simulink model "ctrl_student_HIL"  (R2015a)
settings: Solver=ode4  StartTime=0.0  StopTime=inf  FixedStep=0.01  RelTol=1e-3
(part 1 of 3)
settings Model: CovSFcnEnable=off  Creator=mclab  LastModifiedBy=MCLab
settings DebuggingCC: SolverPrmCheckMsg=warning  InheritedTsInSrcMsg=none
settings RTWCC: SystemTargetFile=NIVeriStand_VxWorks.tlc  TemplateMakefile=NIVeriStand_VxWorks.tmf  Description=NI VeriStand VxWorks Real-Time Target for Release 2007b or later
settings STFCustomTargetCC: GenerateSampleERTMain=off  GeneratePreprocessorConditionals=Disable all  ERTCustomFileBanners=off  MatFileLogging=on  SupportNonInlinedSFcns=on  SupportVariableSizeSignals=off  MATLABClassNameForMDSCustomization=Simulink.SoftwareTarget.TargetSpecificTriggerConfigurationBase  GRTInterface=on  SystemTargetFile=NIVeriStand_VxWorks.tlc

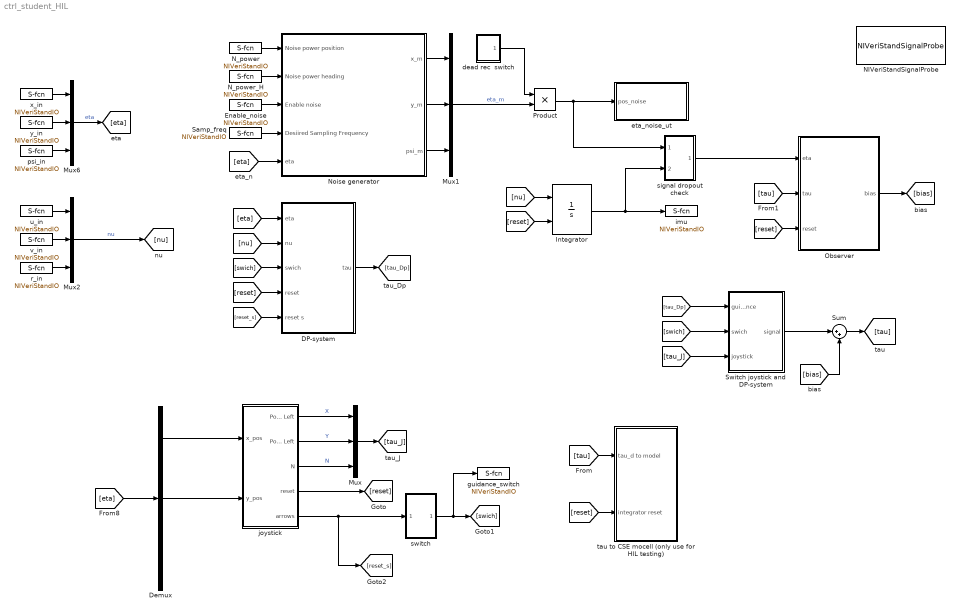
== system ctrl_student_HIL ==
  DP-system : Subsystem
  Demux : Demux  Outputs=3
  Enable_noise : S-Function  Priority=10  FunctionName=NIVeriStandIO  Parameters=width dtype portnum stime stype btype  mask(NI VeriStand Inport){portnum=10, width=-1, stime=-1, dtype=auto, stype=auto, btype=1}
      mask prompts: portnum "Port number:"; width "Port dimensions (-1 for dynamically sized):"; stime "Sample time (-1 for inherited):"; dtype "Data type:"; stype "Signal type:"; btype "Block type:"
      mask help: Use this inport on any level of nested subsystems to allow NI VeriStand software to map signals to it.
      mask init:
      | NIVeriStandIO_init;
      settings: CopyFcn=NIVeriStand_MDL_functions('', 'IO_copy');  DeleteFcn=NIVeriStand_MDL_functions('', 'IO_delete');  MoveFcn=set_param(gcb, 'Mask', 'on');
      mask Callback portnum: NIVeriStand_MDL_functions('', 'IO_setportnum');
      mask TypeOptions dtype: auto | double | single | int8 | uint8 | int16 | uint16 | int32 | uint32 | boolean
      mask Callback dtype: NIVeriStand_MDL_functions('', 'IO_booleansignal');
      mask TypeOptions stype: auto | real | complex
      mask Display:
      | patch([-x x], [-y y], [.90980 .81960 .32156]);
      | plot([xrad -x x xrad], [yrad -y y yrad]);
      | fprintf('NI In%d', portnum);
  Integrator : Integrator  ExternalReset=either
  Mux{,1..2,6} (4 alike) : Mux  Inputs=3
  NIVeriStandSignalProbe : S-Function  FunctionName=NIVeriStandSignalProbe  Parameters=1
  N_power : S-Function  Priority=7  FunctionName=NIVeriStandIO  Parameters=width dtype portnum stime stype btype  mask(NI VeriStand Inport){portnum=7, width=-1, stime=-1, dtype=auto, stype=auto, btype=1}
      mask prompts: portnum "Port number:"; width "Port dimensions (-1 for dynamically sized):"; stime "Sample time (-1 for inherited):"; dtype "Data type:"; stype "Signal type:"; btype "Block type:"
      mask help: Use this inport on any level of nested subsystems to allow NI VeriStand software to map signals to it.
      mask init:
      | NIVeriStandIO_init;
      settings: CopyFcn=NIVeriStand_MDL_functions('', 'IO_copy');  DeleteFcn=NIVeriStand_MDL_functions('', 'IO_delete');  MoveFcn=set_param(gcb, 'Mask', 'on');
      mask Callback portnum: NIVeriStand_MDL_functions('', 'IO_setportnum');
      mask TypeOptions dtype: auto | double | single | int8 | uint8 | int16 | uint16 | int32 | uint32 | boolean
      mask Callback dtype: NIVeriStand_MDL_functions('', 'IO_booleansignal');
      mask TypeOptions stype: auto | real | complex
      mask Display:
      | patch([-x x], [-y y], [.90980 .81960 .32156]);
      | plot([xrad -x x xrad], [yrad -y y yrad]);
      | fprintf('NI In%d', portnum);
  N_power_H : S-Function  Priority=8  FunctionName=NIVeriStandIO  Parameters=width dtype portnum stime stype btype  mask(NI VeriStand Inport){portnum=8, width=-1, stime=-1, dtype=auto, stype=auto, btype=1}
      mask prompts: portnum "Port number:"; width "Port dimensions (-1 for dynamically sized):"; stime "Sample time (-1 for inherited):"; dtype "Data type:"; stype "Signal type:"; btype "Block type:"
      mask help: Use this inport on any level of nested subsystems to allow NI VeriStand software to map signals to it.
      mask init:
      | NIVeriStandIO_init;
      settings: CopyFcn=NIVeriStand_MDL_functions('', 'IO_copy');  DeleteFcn=NIVeriStand_MDL_functions('', 'IO_delete');  MoveFcn=set_param(gcb, 'Mask', 'on');
      mask Callback portnum: NIVeriStand_MDL_functions('', 'IO_setportnum');
      mask TypeOptions dtype: auto | double | single | int8 | uint8 | int16 | uint16 | int32 | uint32 | boolean
      mask Callback dtype: NIVeriStand_MDL_functions('', 'IO_booleansignal');
      mask TypeOptions stype: auto | real | complex
      mask Display:
      | patch([-x x], [-y y], [.90980 .81960 .32156]);
      | plot([xrad -x x xrad], [yrad -y y yrad]);
      | fprintf('NI In%d', portnum);
  Noise generator : Subsystem
  Observer : Subsystem
  Product : Product
  Samp_freq : S-Function  Priority=9  FunctionName=NIVeriStandIO  Parameters=width dtype portnum stime stype btype  mask(NI VeriStand Inport){portnum=9, width=-1, stime=-1, dtype=auto, stype=auto, btype=1}
      mask prompts: portnum "Port number:"; width "Port dimensions (-1 for dynamically sized):"; stime "Sample time (-1 for inherited):"; dtype "Data type:"; stype "Signal type:"; btype "Block type:"
      mask help: Use this inport on any level of nested subsystems to allow NI VeriStand software to map signals to it.
      mask init:
      | NIVeriStandIO_init;
      settings: CopyFcn=NIVeriStand_MDL_functions('', 'IO_copy');  DeleteFcn=NIVeriStand_MDL_functions('', 'IO_delete');  MoveFcn=set_param(gcb, 'Mask', 'on');
      mask Callback portnum: NIVeriStand_MDL_functions('', 'IO_setportnum');
      mask TypeOptions dtype: auto | double | single | int8 | uint8 | int16 | uint16 | int32 | uint32 | boolean
      mask Callback dtype: NIVeriStand_MDL_functions('', 'IO_booleansignal');
      mask TypeOptions stype: auto | real | complex
      mask Display:
      | patch([-x x], [-y y], [.90980 .81960 .32156]);
      | plot([xrad -x x xrad], [yrad -y y yrad]);
      | fprintf('NI In%d', portnum);
  Sum : Sum  Inputs=|++
  Switch joystick and DP-system : MATLAB Function  TreatAsAtomicUnit=on
  dead rec  switch : Subsystem
  eta_noise_ut : Subsystem
  guidance_switch : S-Function  Priority=2  FunctionName=NIVeriStandIO  Parameters=width dtype portnum stime stype btype  mask(NI VeriStand Outport){portnum=2, width=-1, stime=-1, dtype=auto, stype=auto, btype=0}
      mask prompts: portnum "Port number:"; width "Port dimensions (-1 for dynamically sized):"; stime "Sample time (-1 for inherited):"; dtype "Data type:"; stype "Signal type:"; btype "Block type:"
      mask help: Use this outport on any level of nested subsystems to allow NI VeriStand software to map signals to it.
      mask init:
      | NIVeriStandIO_init;
      settings: CopyFcn=NIVeriStand_MDL_functions('', 'IO_copy');  DeleteFcn=NIVeriStand_MDL_functions('', 'IO_delete');  MoveFcn=set_param(gcb, 'Mask', 'on');
      mask Callback portnum: NIVeriStand_MDL_functions('', 'IO_setportnum');
      mask TypeOptions dtype: auto | double | single | int8 | uint8 | int16 | uint16 | int32 | uint32 | boolean
      mask Callback dtype: NIVeriStand_MDL_functions('', 'IO_booleansignal');
      mask TypeOptions stype: auto | real | complex
      mask Display:
      | patch([-x x], [-y y], [.90980 .81960 .32156]);
      | plot([xrad -x x xrad], [yrad -y y yrad]);
      | fprintf('NI Out%d', portnum);
  imu : S-Function  Priority=1  FunctionName=NIVeriStandIO  Parameters=width dtype portnum stime stype btype  mask(NI VeriStand Outport){portnum=1, width=-1, stime=-1, dtype=auto, stype=auto, btype=0}
      mask prompts: portnum "Port number:"; width "Port dimensions (-1 for dynamically sized):"; stime "Sample time (-1 for inherited):"; dtype "Data type:"; stype "Signal type:"; btype "Block type:"
      mask help: Use this outport on any level of nested subsystems to allow NI VeriStand software to map signals to it.
      mask init:
      | NIVeriStandIO_init;
      settings: CopyFcn=NIVeriStand_MDL_functions('', 'IO_copy');  DeleteFcn=NIVeriStand_MDL_functions('', 'IO_delete');  MoveFcn=set_param(gcb, 'Mask', 'on');
      mask Callback portnum: NIVeriStand_MDL_functions('', 'IO_setportnum');
      mask TypeOptions dtype: auto | double | single | int8 | uint8 | int16 | uint16 | int32 | uint32 | boolean
      mask Callback dtype: NIVeriStand_MDL_functions('', 'IO_booleansignal');
      mask TypeOptions stype: auto | real | complex
      mask Display:
      | patch([-x x], [-y y], [.90980 .81960 .32156]);
      | plot([xrad -x x xrad], [yrad -y y yrad]);
      | fprintf('NI Out%d', portnum);
  joystick : Subsystem
  psi_in : S-Function  Priority=2  FunctionName=NIVeriStandIO  Parameters=width dtype portnum stime stype btype  mask(NI VeriStand Inport){portnum=2, width=-1, stime=-1, dtype=auto, stype=auto, btype=1}
      mask prompts: portnum "Port number:"; width "Port dimensions (-1 for dynamically sized):"; stime "Sample time (-1 for inherited):"; dtype "Data type:"; stype "Signal type:"; btype "Block type:"
      mask help: Use this inport on any level of nested subsystems to allow NI VeriStand software to map signals to it.
      mask init:
      | NIVeriStandIO_init;
      settings: CopyFcn=NIVeriStand_MDL_functions('', 'IO_copy');  DeleteFcn=NIVeriStand_MDL_functions('', 'IO_delete');  MoveFcn=set_param(gcb, 'Mask', 'on');
      mask Callback portnum: NIVeriStand_MDL_functions('', 'IO_setportnum');
      mask TypeOptions dtype: auto | double | single | int8 | uint8 | int16 | uint16 | int32 | uint32 | boolean
      mask Callback dtype: NIVeriStand_MDL_functions('', 'IO_booleansignal');
      mask TypeOptions stype: auto | real | complex
      mask Display:
      | patch([-x x], [-y y], [.90980 .81960 .32156]);
      | plot([xrad -x x xrad], [yrad -y y yrad]);
      | fprintf('NI In%d', portnum);
  r_in : S-Function  Priority=4  FunctionName=NIVeriStandIO  Parameters=width dtype portnum stime stype btype  mask(NI VeriStand Inport){portnum=4, width=-1, stime=-1, dtype=auto, stype=auto, btype=1}
      mask prompts: portnum "Port number:"; width "Port dimensions (-1 for dynamically sized):"; stime "Sample time (-1 for inherited):"; dtype "Data type:"; stype "Signal type:"; btype "Block type:"
      mask help: Use this inport on any level of nested subsystems to allow NI VeriStand software to map signals to it.
      mask init:
      | NIVeriStandIO_init;
      settings: CopyFcn=NIVeriStand_MDL_functions('', 'IO_copy');  DeleteFcn=NIVeriStand_MDL_functions('', 'IO_delete');  MoveFcn=set_param(gcb, 'Mask', 'on');
      mask Callback portnum: NIVeriStand_MDL_functions('', 'IO_setportnum');
      mask TypeOptions dtype: auto | double | single | int8 | uint8 | int16 | uint16 | int32 | uint32 | boolean
      mask Callback dtype: NIVeriStand_MDL_functions('', 'IO_booleansignal');
      mask TypeOptions stype: auto | real | complex
      mask Display:
      | patch([-x x], [-y y], [.90980 .81960 .32156]);
      | plot([xrad -x x xrad], [yrad -y y yrad]);
      | fprintf('NI In%d', portnum);
  "signal dropout check " : Subsystem
  switch : Subsystem
  tau to CSE mocell (only use for HIL testing) : Subsystem
  u_in : S-Function  Priority=5  FunctionName=NIVeriStandIO  Parameters=width dtype portnum stime stype btype  mask(NI VeriStand Inport){portnum=5, width=-1, stime=-1, dtype=auto, stype=auto, btype=1}
      mask prompts: portnum "Port number:"; width "Port dimensions (-1 for dynamically sized):"; stime "Sample time (-1 for inherited):"; dtype "Data type:"; stype "Signal type:"; btype "Block type:"
      mask help: Use this inport on any level of nested subsystems to allow NI VeriStand software to map signals to it.
      mask init:
      | NIVeriStandIO_init;
      settings: CopyFcn=NIVeriStand_MDL_functions('', 'IO_copy');  DeleteFcn=NIVeriStand_MDL_functions('', 'IO_delete');  MoveFcn=set_param(gcb, 'Mask', 'on');
      mask Callback portnum: NIVeriStand_MDL_functions('', 'IO_setportnum');
      mask TypeOptions dtype: auto | double | single | int8 | uint8 | int16 | uint16 | int32 | uint32 | boolean
      mask Callback dtype: NIVeriStand_MDL_functions('', 'IO_booleansignal');
      mask TypeOptions stype: auto | real | complex
      mask Display:
      | patch([-x x], [-y y], [.90980 .81960 .32156]);
      | plot([xrad -x x xrad], [yrad -y y yrad]);
      | fprintf('NI In%d', portnum);
  v_in : S-Function  Priority=6  FunctionName=NIVeriStandIO  Parameters=width dtype portnum stime stype btype  mask(NI VeriStand Inport){portnum=6, width=-1, stime=-1, dtype=auto, stype=auto, btype=1}
      mask prompts: portnum "Port number:"; width "Port dimensions (-1 for dynamically sized):"; stime "Sample time (-1 for inherited):"; dtype "Data type:"; stype "Signal type:"; btype "Block type:"
      mask help: Use this inport on any level of nested subsystems to allow NI VeriStand software to map signals to it.
      mask init:
      | NIVeriStandIO_init;
      settings: CopyFcn=NIVeriStand_MDL_functions('', 'IO_copy');  DeleteFcn=NIVeriStand_MDL_functions('', 'IO_delete');  MoveFcn=set_param(gcb, 'Mask', 'on');
      mask Callback portnum: NIVeriStand_MDL_functions('', 'IO_setportnum');
      mask TypeOptions dtype: auto | double | single | int8 | uint8 | int16 | uint16 | int32 | uint32 | boolean
      mask Callback dtype: NIVeriStand_MDL_functions('', 'IO_booleansignal');
      mask TypeOptions stype: auto | real | complex
      mask Display:
      | patch([-x x], [-y y], [.90980 .81960 .32156]);
      | plot([xrad -x x xrad], [yrad -y y yrad]);
      | fprintf('NI In%d', portnum);
  x_in : S-Function  Priority=3  FunctionName=NIVeriStandIO  Parameters=width dtype portnum stime stype btype  mask(NI VeriStand Inport){portnum=3, width=-1, stime=-1, dtype=auto, stype=auto, btype=1}
      mask prompts: portnum "Port number:"; width "Port dimensions (-1 for dynamically sized):"; stime "Sample time (-1 for inherited):"; dtype "Data type:"; stype "Signal type:"; btype "Block type:"
      mask help: Use this inport on any level of nested subsystems to allow NI VeriStand software to map signals to it.
      mask init:
      | NIVeriStandIO_init;
      settings: CopyFcn=NIVeriStand_MDL_functions('', 'IO_copy');  DeleteFcn=NIVeriStand_MDL_functions('', 'IO_delete');  MoveFcn=set_param(gcb, 'Mask', 'on');
      mask Callback portnum: NIVeriStand_MDL_functions('', 'IO_setportnum');
      mask TypeOptions dtype: auto | double | single | int8 | uint8 | int16 | uint16 | int32 | uint32 | boolean
      mask Callback dtype: NIVeriStand_MDL_functions('', 'IO_booleansignal');
      mask TypeOptions stype: auto | real | complex
      mask Display:
      | patch([-x x], [-y y], [.90980 .81960 .32156]);
      | plot([xrad -x x xrad], [yrad -y y yrad]);
      | fprintf('NI In%d', portnum);
  y_in : S-Function  Priority=1  FunctionName=NIVeriStandIO  Parameters=width dtype portnum stime stype btype  mask(NI VeriStand Inport){portnum=1, width=-1, stime=-1, dtype=auto, stype=auto, btype=1}
      mask prompts: portnum "Port number:"; width "Port dimensions (-1 for dynamically sized):"; stime "Sample time (-1 for inherited):"; dtype "Data type:"; stype "Signal type:"; btype "Block type:"
      mask help: Use this inport on any level of nested subsystems to allow NI VeriStand software to map signals to it.
      mask init:
      | NIVeriStandIO_init;
      settings: CopyFcn=NIVeriStand_MDL_functions('', 'IO_copy');  DeleteFcn=NIVeriStand_MDL_functions('', 'IO_delete');  MoveFcn=set_param(gcb, 'Mask', 'on');
      mask Callback portnum: NIVeriStand_MDL_functions('', 'IO_setportnum');
      mask TypeOptions dtype: auto | double | single | int8 | uint8 | int16 | uint16 | int32 | uint32 | boolean
      mask Callback dtype: NIVeriStand_MDL_functions('', 'IO_booleansignal');
      mask TypeOptions stype: auto | real | complex
      mask Display:
      | patch([-x x], [-y y], [.90980 .81960 .32156]);
      | plot([xrad -x x xrad], [yrad -y y yrad]);
      | fprintf('NI In%d', portnum);
  wires:
  joystick/3(N) -> Mux/3  "N"
  x_in/1 -> Mux6/1
  y_in/1 -> Mux6/2
  psi_in/1 -> Mux6/3
  Noise generator/1(x_m) -> Mux1/1
  Noise generator/2(y_m) -> Mux1/2
  Noise generator/3(psi_m) -> Mux1/3
  joystick/2(PosY Left) -> Mux/2  "Y"
  joystick/1(PosX Left) -> Mux/1  "X"
  u_in/1 -> Mux2/1
  v_in/1 -> Mux2/2
  r_in/1 -> Mux2/3
  Samp_freq/1 -> Noise generator/4(Desiired Sampling Frequency)
  Enable_noise/1 -> Noise generator/3(Enable noise)
  N_power_H/1 -> Noise generator/2(Noise power heading)
  N_power/1 -> Noise generator/1(Noise power position)
  Mux1/1 -> Product/2  "eta_m"
  Product/1 -> eta_noise_ut/1(pos_noise), "signal dropout check "/1(eta_n)
  dead rec  switch/1(Out1) -> Product/1
  "signal dropout check "/1(eta) -> Observer/1(eta)
  joystick/4(reset) -> [reset]
  [reset] -> Observer/3(reset)
  [reset] -> tau to CSE mocell (only use for HIL testing)/2(integrator reset)
  Integrator/1 -> imu/1, "signal dropout check "/2(imu)
  [reset] -> Integrator/2
  joystick/5(arrows) -> [reset_s], switch/1(In1)
  switch/1(Out1) -> guidance_switch/1, [swich]
  [swich] -> DP-system/3(swich)
  [swich] -> Switch joystick and DP-system/2(swich)
  [reset] -> DP-system/4("reset ")
  [reset_s] -> DP-system/5(reset s)
  [eta] -> Noise generator/5(eta)
  [eta] -> DP-system/1(eta)
  [eta] -> Demux/1
  Demux/1 -> joystick/1(x_pos)
  Demux/2 -> joystick/2(y_pos)
  Mux6/1 -> [eta]  "eta"
  Mux2/1 -> [nu]  "nu"
  [nu] -> DP-system/2(nu)
  [nu] -> Integrator/1
  DP-system/1(tau) -> [tau_Dp]
  [tau_Dp] -> Switch joystick and DP-system/1(guidance)
  Mux/1 -> [tau_J]
  [tau_J] -> Switch joystick and DP-system/3(joystick)
  [tau] -> Observer/2(tau)
  [tau] -> tau to CSE mocell (only use for HIL testing)/1(tau_d to model)
  Observer/1(bias) -> [bias]
  Switch joystick and DP-system/1(signal) -> Sum/1
  [bias] -> Sum/2
  Sum/1 -> [tau]

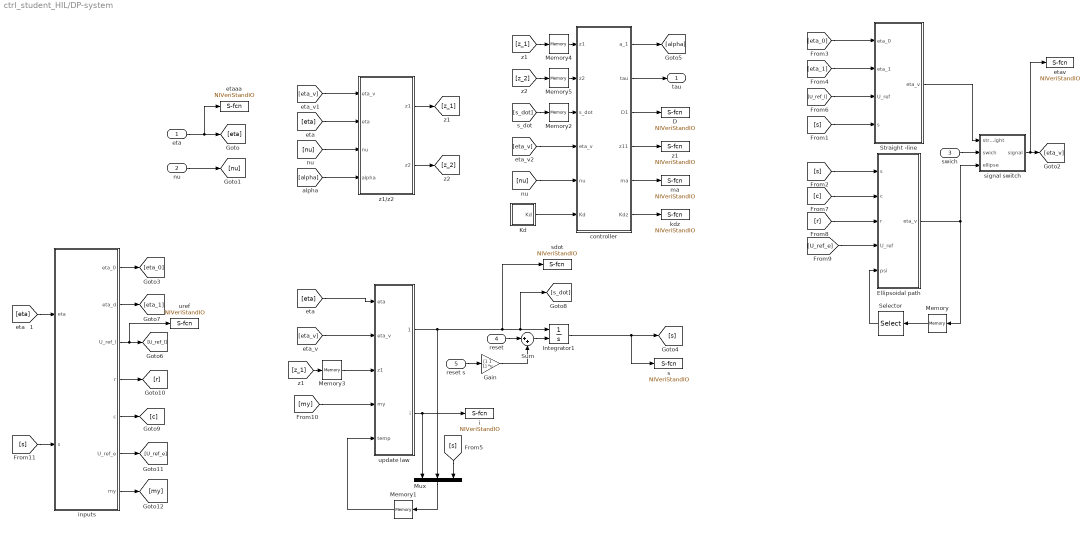
== system ctrl_student_HIL/DP-system ==
  eta : Inport
  nu : Inport  Port=2
  swich : Inport  Port=3
  "reset " : Inport  Port=4
  reset s : Inport  Port=5
  D : S-Function  Priority=2  FunctionName=NIVeriStandIO  Parameters=width dtype portnum stime stype btype  mask(NI VeriStand Outport){portnum=2, width=-1, stime=-1, dtype=auto, stype=auto, btype=0}
      mask prompts: portnum "Port number:"; width "Port dimensions (-1 for dynamically sized):"; stime "Sample time (-1 for inherited):"; dtype "Data type:"; stype "Signal type:"; btype "Block type:"
      mask help: Use this outport on any level of nested subsystems to allow NI VeriStand software to map signals to it.
      mask init:
      | NIVeriStandIO_init;
      settings: CopyFcn=NIVeriStand_MDL_functions('', 'IO_copy');  DeleteFcn=NIVeriStand_MDL_functions('', 'IO_delete');  MoveFcn=set_param(gcb, 'Mask', 'on');
      mask Callback portnum: NIVeriStand_MDL_functions('', 'IO_setportnum');
      mask TypeOptions dtype: auto | double | single | int8 | uint8 | int16 | uint16 | int32 | uint32 | boolean
      mask Callback dtype: NIVeriStand_MDL_functions('', 'IO_booleansignal');
      mask TypeOptions stype: auto | real | complex
      mask Display:
      | patch([-x x], [-y y], [.90980 .81960 .32156]);
      | plot([xrad -x x xrad], [yrad -y y yrad]);
      | fprintf('NI Out%d', portnum);
  Ellipsoidal path : MATLAB Function  TreatAsAtomicUnit=on
  Gain : Gain  Gain=[1 1 1]  Multiplication=Matrix(K*u)
  Integrator1 : Integrator  ExternalReset=either
  Kd : Subsystem
  Memory : Memory
  Memory1 : Memory  X0=[0 0 0]
  Memory2 : Memory
  Memory3 : Memory
  Memory4 : Memory  X0=[0;0;0]
  Memory5 : Memory  X0=[0;0;0]
  Mux : Mux  Inputs=3
  Selector : Selector  InputPortWidth=11  Indices=[3]
  "Straight -line " : MATLAB Function  TreatAsAtomicUnit=on
  Sum : Sum  Inputs=|++
  controller : MATLAB Function  TreatAsAtomicUnit=on
  etaaa : S-Function  Priority=6  FunctionName=NIVeriStandIO  Parameters=width dtype portnum stime stype btype  mask(NI VeriStand Outport){portnum=6, width=-1, stime=-1, dtype=auto, stype=auto, btype=0}
      mask prompts: portnum "Port number:"; width "Port dimensions (-1 for dynamically sized):"; stime "Sample time (-1 for inherited):"; dtype "Data type:"; stype "Signal type:"; btype "Block type:"
      mask help: Use this outport on any level of nested subsystems to allow NI VeriStand software to map signals to it.
      mask init:
      | NIVeriStandIO_init;
      settings: CopyFcn=NIVeriStand_MDL_functions('', 'IO_copy');  DeleteFcn=NIVeriStand_MDL_functions('', 'IO_delete');  MoveFcn=set_param(gcb, 'Mask', 'on');
      mask Callback portnum: NIVeriStand_MDL_functions('', 'IO_setportnum');
      mask TypeOptions dtype: auto | double | single | int8 | uint8 | int16 | uint16 | int32 | uint32 | boolean
      mask Callback dtype: NIVeriStand_MDL_functions('', 'IO_booleansignal');
      mask TypeOptions stype: auto | real | complex
      mask Display:
      | patch([-x x], [-y y], [.90980 .81960 .32156]);
      | plot([xrad -x x xrad], [yrad -y y yrad]);
      | fprintf('NI Out%d', portnum);
  etav : S-Function  Priority=7  FunctionName=NIVeriStandIO  Parameters=width dtype portnum stime stype btype  mask(NI VeriStand Outport){portnum=7, width=-1, stime=-1, dtype=auto, stype=auto, btype=0}
      mask prompts: portnum "Port number:"; width "Port dimensions (-1 for dynamically sized):"; stime "Sample time (-1 for inherited):"; dtype "Data type:"; stype "Signal type:"; btype "Block type:"
      mask help: Use this outport on any level of nested subsystems to allow NI VeriStand software to map signals to it.
      mask init:
      | NIVeriStandIO_init;
      settings: CopyFcn=NIVeriStand_MDL_functions('', 'IO_copy');  DeleteFcn=NIVeriStand_MDL_functions('', 'IO_delete');  MoveFcn=set_param(gcb, 'Mask', 'on');
      mask Callback portnum: NIVeriStand_MDL_functions('', 'IO_setportnum');
      mask TypeOptions dtype: auto | double | single | int8 | uint8 | int16 | uint16 | int32 | uint32 | boolean
      mask Callback dtype: NIVeriStand_MDL_functions('', 'IO_booleansignal');
      mask TypeOptions stype: auto | real | complex
      mask Display:
      | patch([-x x], [-y y], [.90980 .81960 .32156]);
      | plot([xrad -x x xrad], [yrad -y y yrad]);
      | fprintf('NI Out%d', portnum);
  i : S-Function  Priority=10  FunctionName=NIVeriStandIO  Parameters=width dtype portnum stime stype btype  mask(NI VeriStand Outport){portnum=10, width=-1, stime=-1, dtype=auto, stype=auto, btype=0}
      mask prompts: portnum "Port number:"; width "Port dimensions (-1 for dynamically sized):"; stime "Sample time (-1 for inherited):"; dtype "Data type:"; stype "Signal type:"; btype "Block type:"
      mask help: Use this outport on any level of nested subsystems to allow NI VeriStand software to map signals to it.
      mask init:
      | NIVeriStandIO_init;
      settings: CopyFcn=NIVeriStand_MDL_functions('', 'IO_copy');  DeleteFcn=NIVeriStand_MDL_functions('', 'IO_delete');  MoveFcn=set_param(gcb, 'Mask', 'on');
      mask Callback portnum: NIVeriStand_MDL_functions('', 'IO_setportnum');
      mask TypeOptions dtype: auto | double | single | int8 | uint8 | int16 | uint16 | int32 | uint32 | boolean
      mask Callback dtype: NIVeriStand_MDL_functions('', 'IO_booleansignal');
      mask TypeOptions stype: auto | real | complex
      mask Display:
      | patch([-x x], [-y y], [.90980 .81960 .32156]);
      | plot([xrad -x x xrad], [yrad -y y yrad]);
      | fprintf('NI Out%d', portnum);
  inputs : MATLAB Function  TreatAsAtomicUnit=on
  kdz : S-Function  Priority=5  FunctionName=NIVeriStandIO  Parameters=width dtype portnum stime stype btype  mask(NI VeriStand Outport){portnum=5, width=-1, stime=-1, dtype=auto, stype=auto, btype=0}
      mask prompts: portnum "Port number:"; width "Port dimensions (-1 for dynamically sized):"; stime "Sample time (-1 for inherited):"; dtype "Data type:"; stype "Signal type:"; btype "Block type:"
      mask help: Use this outport on any level of nested subsystems to allow NI VeriStand software to map signals to it.
      mask init:
      | NIVeriStandIO_init;
      settings: CopyFcn=NIVeriStand_MDL_functions('', 'IO_copy');  DeleteFcn=NIVeriStand_MDL_functions('', 'IO_delete');  MoveFcn=set_param(gcb, 'Mask', 'on');
      mask Callback portnum: NIVeriStand_MDL_functions('', 'IO_setportnum');
      mask TypeOptions dtype: auto | double | single | int8 | uint8 | int16 | uint16 | int32 | uint32 | boolean
      mask Callback dtype: NIVeriStand_MDL_functions('', 'IO_booleansignal');
      mask TypeOptions stype: auto | real | complex
      mask Display:
      | patch([-x x], [-y y], [.90980 .81960 .32156]);
      | plot([xrad -x x xrad], [yrad -y y yrad]);
      | fprintf('NI Out%d', portnum);
  ma : S-Function  Priority=4  FunctionName=NIVeriStandIO  Parameters=width dtype portnum stime stype btype  mask(NI VeriStand Outport){portnum=4, width=-1, stime=-1, dtype=auto, stype=auto, btype=0}
      mask prompts: portnum "Port number:"; width "Port dimensions (-1 for dynamically sized):"; stime "Sample time (-1 for inherited):"; dtype "Data type:"; stype "Signal type:"; btype "Block type:"
      mask help: Use this outport on any level of nested subsystems to allow NI VeriStand software to map signals to it.
      mask init:
      | NIVeriStandIO_init;
      settings: CopyFcn=NIVeriStand_MDL_functions('', 'IO_copy');  DeleteFcn=NIVeriStand_MDL_functions('', 'IO_delete');  MoveFcn=set_param(gcb, 'Mask', 'on');
      mask Callback portnum: NIVeriStand_MDL_functions('', 'IO_setportnum');
      mask TypeOptions dtype: auto | double | single | int8 | uint8 | int16 | uint16 | int32 | uint32 | boolean
      mask Callback dtype: NIVeriStand_MDL_functions('', 'IO_booleansignal');
      mask TypeOptions stype: auto | real | complex
      mask Display:
      | patch([-x x], [-y y], [.90980 .81960 .32156]);
      | plot([xrad -x x xrad], [yrad -y y yrad]);
      | fprintf('NI Out%d', portnum);
  s : S-Function  Priority=1  FunctionName=NIVeriStandIO  Parameters=width dtype portnum stime stype btype  mask(NI VeriStand Outport){portnum=1, width=-1, stime=-1, dtype=auto, stype=auto, btype=0}
      mask prompts: portnum "Port number:"; width "Port dimensions (-1 for dynamically sized):"; stime "Sample time (-1 for inherited):"; dtype "Data type:"; stype "Signal type:"; btype "Block type:"
      mask help: Use this outport on any level of nested subsystems to allow NI VeriStand software to map signals to it.
      mask init:
      | NIVeriStandIO_init;
      settings: CopyFcn=NIVeriStand_MDL_functions('', 'IO_copy');  DeleteFcn=NIVeriStand_MDL_functions('', 'IO_delete');  MoveFcn=set_param(gcb, 'Mask', 'on');
      mask Callback portnum: NIVeriStand_MDL_functions('', 'IO_setportnum');
      mask TypeOptions dtype: auto | double | single | int8 | uint8 | int16 | uint16 | int32 | uint32 | boolean
      mask Callback dtype: NIVeriStand_MDL_functions('', 'IO_booleansignal');
      mask TypeOptions stype: auto | real | complex
      mask Display:
      | patch([-x x], [-y y], [.90980 .81960 .32156]);
      | plot([xrad -x x xrad], [yrad -y y yrad]);
      | fprintf('NI Out%d', portnum);
  sdot : S-Function  Priority=9  FunctionName=NIVeriStandIO  Parameters=width dtype portnum stime stype btype  mask(NI VeriStand Outport){portnum=9, width=-1, stime=-1, dtype=auto, stype=auto, btype=0}
      mask prompts: portnum "Port number:"; width "Port dimensions (-1 for dynamically sized):"; stime "Sample time (-1 for inherited):"; dtype "Data type:"; stype "Signal type:"; btype "Block type:"
      mask help: Use this outport on any level of nested subsystems to allow NI VeriStand software to map signals to it.
      mask init:
      | NIVeriStandIO_init;
      settings: CopyFcn=NIVeriStand_MDL_functions('', 'IO_copy');  DeleteFcn=NIVeriStand_MDL_functions('', 'IO_delete');  MoveFcn=set_param(gcb, 'Mask', 'on');
      mask Callback portnum: NIVeriStand_MDL_functions('', 'IO_setportnum');
      mask TypeOptions dtype: auto | double | single | int8 | uint8 | int16 | uint16 | int32 | uint32 | boolean
      mask Callback dtype: NIVeriStand_MDL_functions('', 'IO_booleansignal');
      mask TypeOptions stype: auto | real | complex
      mask Display:
      | patch([-x x], [-y y], [.90980 .81960 .32156]);
      | plot([xrad -x x xrad], [yrad -y y yrad]);
      | fprintf('NI Out%d', portnum);
  "signal switch " : MATLAB Function  TreatAsAtomicUnit=on
  update law : MATLAB Function  TreatAsAtomicUnit=on
  "uref " : S-Function  Priority=8  FunctionName=NIVeriStandIO  Parameters=width dtype portnum stime stype btype  mask(NI VeriStand Outport){portnum=8, width=-1, stime=-1, dtype=auto, stype=auto, btype=0}
      mask prompts: portnum "Port number:"; width "Port dimensions (-1 for dynamically sized):"; stime "Sample time (-1 for inherited):"; dtype "Data type:"; stype "Signal type:"; btype "Block type:"
      mask help: Use this outport on any level of nested subsystems to allow NI VeriStand software to map signals to it.
      mask init:
      | NIVeriStandIO_init;
      settings: CopyFcn=NIVeriStand_MDL_functions('', 'IO_copy');  DeleteFcn=NIVeriStand_MDL_functions('', 'IO_delete');  MoveFcn=set_param(gcb, 'Mask', 'on');
      mask Callback portnum: NIVeriStand_MDL_functions('', 'IO_setportnum');
      mask TypeOptions dtype: auto | double | single | int8 | uint8 | int16 | uint16 | int32 | uint32 | boolean
      mask Callback dtype: NIVeriStand_MDL_functions('', 'IO_booleansignal');
      mask TypeOptions stype: auto | real | complex
      mask Display:
      | patch([-x x], [-y y], [.90980 .81960 .32156]);
      | plot([xrad -x x xrad], [yrad -y y yrad]);
      | fprintf('NI Out%d', portnum);
  z1 : S-Function  Priority=3  FunctionName=NIVeriStandIO  Parameters=width dtype portnum stime stype btype  mask(NI VeriStand Outport){portnum=3, width=-1, stime=-1, dtype=auto, stype=auto, btype=0}
      mask prompts: portnum "Port number:"; width "Port dimensions (-1 for dynamically sized):"; stime "Sample time (-1 for inherited):"; dtype "Data type:"; stype "Signal type:"; btype "Block type:"
      mask help: Use this outport on any level of nested subsystems to allow NI VeriStand software to map signals to it.
      mask init:
      | NIVeriStandIO_init;
      settings: CopyFcn=NIVeriStand_MDL_functions('', 'IO_copy');  DeleteFcn=NIVeriStand_MDL_functions('', 'IO_delete');  MoveFcn=set_param(gcb, 'Mask', 'on');
      mask Callback portnum: NIVeriStand_MDL_functions('', 'IO_setportnum');
      mask TypeOptions dtype: auto | double | single | int8 | uint8 | int16 | uint16 | int32 | uint32 | boolean
      mask Callback dtype: NIVeriStand_MDL_functions('', 'IO_booleansignal');
      mask TypeOptions stype: auto | real | complex
      mask Display:
      | patch([-x x], [-y y], [.90980 .81960 .32156]);
      | plot([xrad -x x xrad], [yrad -y y yrad]);
      | fprintf('NI Out%d', portnum);
  z1/z2 : MATLAB Function  TreatAsAtomicUnit=on
  tau : Outport
  wires:
  nu/1 -> [nu]
  [eta_0] -> "Straight -line "/1(eta_0)
  [eta_1] -> "Straight -line "/2(eta_1)
  [c] -> Ellipsoidal path/2(c)
  [r] -> Ellipsoidal path/3(r)
  [U_ref_e] -> Ellipsoidal path/4(U_ref)
  [eta] -> z1/z2/2(eta)
  [eta] -> update law/1(eta)
  swich/1 -> "signal switch "/2(swich)
  "signal switch "/1(signal) -> etav/1, [eta_v]
  [eta_v] -> update law/2(eta_v)
  [eta_v] -> z1/z2/1(eta_v)
  [eta_v] -> controller/4(eta_v)
  Integrator1/1 -> [s], s/1
  [my] -> update law/4(my)
  [U_ref_l] -> "Straight -line "/3(U_ref)
  [alpha] -> z1/z2/4(alpha)
  z1/z2/1(z1) -> [z_1]
  z1/z2/2(z2) -> [z_2]
  [s] -> "Straight -line "/4(s)
  [s] -> Ellipsoidal path/1(s)
  [s_dot] -> Memory2/1
  Memory2/1 -> controller/3(s_dot)
  controller/1(a_1) -> [alpha]
  [z_1] -> Memory3/1
  Memory3/1 -> update law/3(z1)
  [z_1] -> Memory4/1
  Memory4/1 -> controller/1(z1)
  [z_2] -> Memory5/1
  inputs/1(eta_0) -> [eta_0]
  inputs/2(eta_d) -> [eta_1]
  inputs/3(U_ref_l) -> "uref "/1, [U_ref_l]
  inputs/5(c) -> [c]
  inputs/4(r) -> [r]
  inputs/6(U_ref_e) -> [U_ref_e]
  inputs/7(my) -> [my]
  [s] -> inputs/2(s)
  "reset "/1 -> Sum/1
  Sum/1 -> Integrator1/2
  reset s/1 -> Gain/1
  Gain/1 -> Sum/2
  controller/3(D1) -> D/1
  controller/4(z11) -> z1/1
  controller/5(ma) -> ma/1
  controller/6(Kdz) -> kdz/1
  controller/2(tau) -> tau/1
  eta/1 -> [eta], etaaa/1
  Memory5/1 -> controller/2(z2)
  Ellipsoidal path/1(eta_v) -> "signal switch "/3(ellipse), Memory/1
  [nu] -> controller/5(nu)
  Kd/1(Kd) -> controller/6(Kd)
  "Straight -line "/1(eta_v) -> "signal switch "/1(straight)
  Selector/1 -> Ellipsoidal path/5(psi)
  Memory/1 -> Selector/1
  [nu] -> z1/z2/3(nu)
  [eta] -> inputs/1(eta)
  update law/1(s_dot1) -> sdot/1, [s_dot], Integrator1/1, Mux/2
  Memory1/1 -> update law/5(temp)
  update law/2(i) -> i/1, Mux/1
  Mux/1 -> Memory1/1
  [s] -> Mux/3

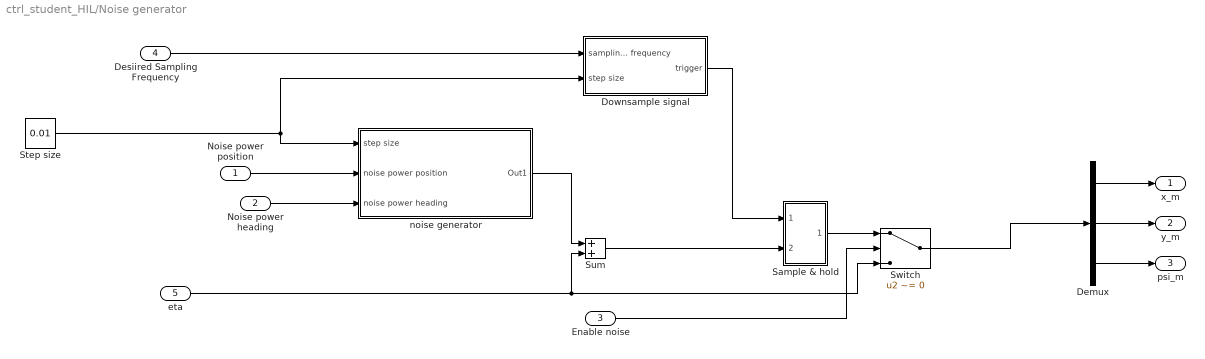
== system ctrl_student_HIL/Noise generator ==
  Noise power position : Inport
  Noise power heading : Inport  Port=2
  Enable noise : Inport  Port=3
  Desiired Sampling Frequency : Inport  Port=4
  eta : Inport  Port=5
  Demux : Demux  Outputs=3
  Downsample	signal : Subsystem
  Sample & hold : Subsystem
  Step size : Constant  Value=0.01
  Sum : Sum
  Switch : Switch  Criteria=u2 ~= 0
  noise generator : Subsystem
  x_m : Outport
  y_m : Outport  Port=2
  psi_m : Outport  Port=3
  wires:
  Step size/1 -> Downsample	signal/2(step size), noise generator/1(step size)
  Downsample	signal/1(trigger) -> Sample & hold/1(trigger)
  Desiired Sampling Frequency/1 -> Downsample	signal/1(sampling frequency)
  eta/1 -> Sum/2, Switch/3
  Sum/1 -> Sample & hold/2(input)
  Sample & hold/1(output) -> Switch/1
  Noise power position/1 -> noise generator/2(noise power position)
  Noise power heading/1 -> noise generator/3(noise power heading)
  noise generator/1(Out1) -> Sum/1
  Enable noise/1 -> Switch/2
  Switch/1 -> Demux/1
  Demux/3 -> psi_m/1
  Demux/2 -> y_m/1
  Demux/1 -> x_m/1

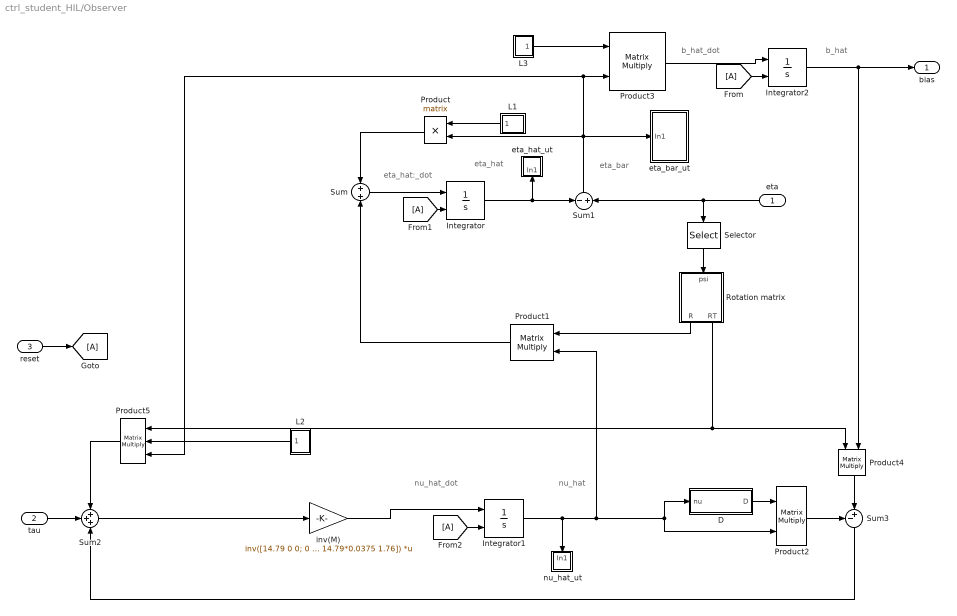
== system ctrl_student_HIL/Observer ==
  note: b_hat
  note: b_hat_dot
  note: eta_bar
  note: nu_hat
  note: nu_hat_dot
  note: eta_hat:_dot
  note: eta_hat
  eta : Inport  PortDimensions=3
  tau : Inport  Port=2  PortDimensions=3
  reset : Inport  Port=3  PortDimensions=1
  D : MATLAB Function  TreatAsAtomicUnit=on
  Integrator : Integrator  ExternalReset=either
  Integrator1 : Integrator  ExternalReset=either
  Integrator2 : Integrator  ExternalReset=either
  L1 : Subsystem
  L2 : Subsystem
  L3 : Subsystem
  Product{,1..4} (5 alike) : Product  Multiplication=Matrix(*)
  Product5 : Product  Inputs=3  Multiplication=Matrix(*)
  Rotation matrix : MATLAB Function  TreatAsAtomicUnit=on
  Selector : Selector  InputPortWidth=3  Indices=[3]
  Sum : Sum
  Sum1 : Sum  Inputs=-+
  Sum2 : Sum  Inputs=+++
  Sum3 : Sum  Inputs=-+|
  eta_bar_ut : Subsystem
  eta_hat_ut : Subsystem
  inv(M) : Gain  Gain=|  Multiplication=Matrix(K*u) (u vector)
      | inv([14.79 0 0;
      | 0 14.79 14.79*0.0375;
      | 0 14.79*0.0375 1.76])
  nu_hat_ut : Subsystem
  bias : Outport
  wires:
  Sum/1 -> Integrator/1
  Integrator/1 -> Sum1/1, eta_hat_ut/1(In1)
  eta/1 -> Selector/1, Sum1/2
  Sum1/1 -> Product5/3, Product3/2, eta_bar_ut/1(In1), Product/2
  L1/1(L1) -> Product/1
  Product/1 -> Sum/1
  Selector/1 -> Rotation matrix/1(psi)
  Integrator1/1 -> nu_hat_ut/1(In1), Product1/2, Product2/2, D/1(nu)
  inv(M)/1 -> Integrator1/1
  Rotation matrix/1(R) -> Product1/1
  Product1/1 -> Sum/2
  D/1(D) -> Product2/1
  Sum2/1 -> inv(M)/1
  Product3/1 -> Integrator2/1
  L3/1(L3) -> Product3/1
  Rotation matrix/2(RT) -> Product4/1, Product5/1
  Product2/1 -> Sum3/1
  Product4/1 -> Sum3/2
  Sum3/1 -> Sum2/3
  L2/1(L2) -> Product5/2
  tau/1 -> Sum2/2
  Product5/1 -> Sum2/1
  reset/1 -> [A]
  [A] -> Integrator2/2
  [A] -> Integrator/2
  [A] -> Integrator1/2
  Integrator2/1 -> bias/1, Product4/2

== system ctrl_student_HIL/dead rec  switch ==
  Constant : Constant  Value=0
  Constant1 : Constant
  Switch1 : Switch  Criteria=u2 ~= 0
  dead : S-Function  Priority=11  FunctionName=NIVeriStandIO  Parameters=width dtype portnum stime stype btype  mask(NI VeriStand Inport){portnum=11, width=-1, stime=-1, dtype=auto, stype=auto, btype=1}
      mask prompts: portnum "Port number:"; width "Port dimensions (-1 for dynamically sized):"; stime "Sample time (-1 for inherited):"; dtype "Data type:"; stype "Signal type:"; btype "Block type:"
      mask help: Use this inport on any level of nested subsystems to allow NI VeriStand software to map signals to it.
      mask init:
      | NIVeriStandIO_init;
      settings: CopyFcn=NIVeriStand_MDL_functions('', 'IO_copy');  DeleteFcn=NIVeriStand_MDL_functions('', 'IO_delete');  MoveFcn=set_param(gcb, 'Mask', 'on');
      mask Callback portnum: NIVeriStand_MDL_functions('', 'IO_setportnum');
      mask TypeOptions dtype: auto | double | single | int8 | uint8 | int16 | uint16 | int32 | uint32 | boolean
      mask Callback dtype: NIVeriStand_MDL_functions('', 'IO_booleansignal');
      mask TypeOptions stype: auto | real | complex
      mask Display:
      | patch([-x x], [-y y], [.90980 .81960 .32156]);
      | plot([xrad -x x xrad], [yrad -y y yrad]);
      | fprintf('NI In%d', portnum);
  Out1 : Outport
  wires:
  Constant/1 -> Switch1/1
  Constant1/1 -> Switch1/3
  dead/1 -> Switch1/2
  Switch1/1 -> Out1/1

== system ctrl_student_HIL/eta_noise_ut ==
  pos_noise : Inport
  Demux1 : Demux  Outputs=3
  psi_noise : S-Function  Priority=1  FunctionName=NIVeriStandIO  Parameters=width dtype portnum stime stype btype  mask(NI VeriStand Outport){portnum=1, width=-1, stime=-1, dtype=auto, stype=auto, btype=0}
      mask prompts: portnum "Port number:"; width "Port dimensions (-1 for dynamically sized):"; stime "Sample time (-1 for inherited):"; dtype "Data type:"; stype "Signal type:"; btype "Block type:"
      mask help: Use this outport on any level of nested subsystems to allow NI VeriStand software to map signals to it.
      mask init:
      | NIVeriStandIO_init;
      settings: CopyFcn=NIVeriStand_MDL_functions('', 'IO_copy');  DeleteFcn=NIVeriStand_MDL_functions('', 'IO_delete');  MoveFcn=set_param(gcb, 'Mask', 'on');
      mask Callback portnum: NIVeriStand_MDL_functions('', 'IO_setportnum');
      mask TypeOptions dtype: auto | double | single | int8 | uint8 | int16 | uint16 | int32 | uint32 | boolean
      mask Callback dtype: NIVeriStand_MDL_functions('', 'IO_booleansignal');
      mask TypeOptions stype: auto | real | complex
      mask Display:
      | patch([-x x], [-y y], [.90980 .81960 .32156]);
      | plot([xrad -x x xrad], [yrad -y y yrad]);
      | fprintf('NI Out%d', portnum);
  x_noise : S-Function  Priority=2  FunctionName=NIVeriStandIO  Parameters=width dtype portnum stime stype btype  mask(NI VeriStand Outport){portnum=2, width=-1, stime=-1, dtype=auto, stype=auto, btype=0}
      mask prompts: portnum "Port number:"; width "Port dimensions (-1 for dynamically sized):"; stime "Sample time (-1 for inherited):"; dtype "Data type:"; stype "Signal type:"; btype "Block type:"
      mask help: Use this outport on any level of nested subsystems to allow NI VeriStand software to map signals to it.
      mask init:
      | NIVeriStandIO_init;
      settings: CopyFcn=NIVeriStand_MDL_functions('', 'IO_copy');  DeleteFcn=NIVeriStand_MDL_functions('', 'IO_delete');  MoveFcn=set_param(gcb, 'Mask', 'on');
      mask Callback portnum: NIVeriStand_MDL_functions('', 'IO_setportnum');
      mask TypeOptions dtype: auto | double | single | int8 | uint8 | int16 | uint16 | int32 | uint32 | boolean
      mask Callback dtype: NIVeriStand_MDL_functions('', 'IO_booleansignal');
      mask TypeOptions stype: auto | real | complex
      mask Display:
      | patch([-x x], [-y y], [.90980 .81960 .32156]);
      | plot([xrad -x x xrad], [yrad -y y yrad]);
      | fprintf('NI Out%d', portnum);
  y_noise : S-Function  Priority=3  FunctionName=NIVeriStandIO  Parameters=width dtype portnum stime stype btype  mask(NI VeriStand Outport){portnum=3, width=-1, stime=-1, dtype=auto, stype=auto, btype=0}
      mask prompts: portnum "Port number:"; width "Port dimensions (-1 for dynamically sized):"; stime "Sample time (-1 for inherited):"; dtype "Data type:"; stype "Signal type:"; btype "Block type:"
      mask help: Use this outport on any level of nested subsystems to allow NI VeriStand software to map signals to it.
      mask init:
      | NIVeriStandIO_init;
      settings: CopyFcn=NIVeriStand_MDL_functions('', 'IO_copy');  DeleteFcn=NIVeriStand_MDL_functions('', 'IO_delete');  MoveFcn=set_param(gcb, 'Mask', 'on');
      mask Callback portnum: NIVeriStand_MDL_functions('', 'IO_setportnum');
      mask TypeOptions dtype: auto | double | single | int8 | uint8 | int16 | uint16 | int32 | uint32 | boolean
      mask Callback dtype: NIVeriStand_MDL_functions('', 'IO_booleansignal');
      mask TypeOptions stype: auto | real | complex
      mask Display:
      | patch([-x x], [-y y], [.90980 .81960 .32156]);
      | plot([xrad -x x xrad], [yrad -y y yrad]);
      | fprintf('NI Out%d', portnum);
  wires:
  Demux1/1 -> x_noise/1
  pos_noise/1 -> Demux1/1
  Demux1/2 -> y_noise/1
  Demux1/3 -> psi_noise/1
